simulink subsystem "MPC"  (R2024a)
settings: Solver=VariableStepAuto  StartTime=0.0  StopTime=10.0  RelTol=1e-3
libraries: mpclib x1
settings Model: Creator=cianc  LastModifiedBy=cianc

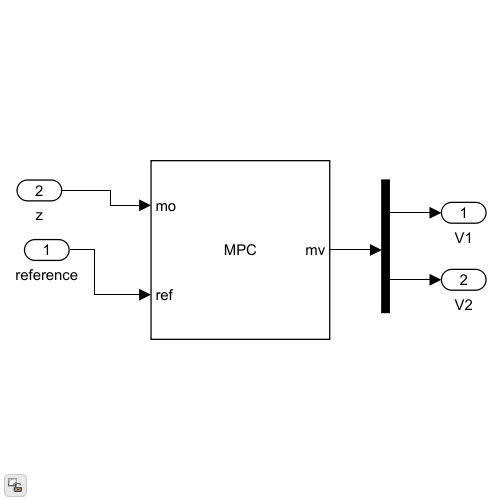
[thumbnail: Simulink's stored preview of the top-level diagram]
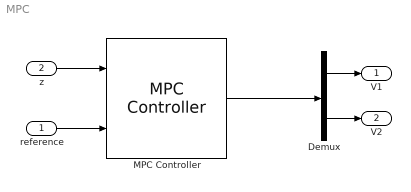
== system MPC ==
  reference : Inport
  z : Inport  Port=2
  Demux : Demux  Outputs=2
  MPC Controller : mpclib/MPC Controller  SCDEnableBlockLinearizationSpecification=on  is_multiple=0  enable_value=0  return_u0=off  updateMPCinCallerWorkspace=on  md_inport=off  mv_inport=off  uref_inport=off  return_cost=off  return_mvseq=off  return_qpstatus=off  return_xseq=off  return_state=off  return_ovseq=off  state_inport=off  umin_inport=off  umax_inport=off  ymin_inport=off  ymax_inport=off  cc_inport=off  ywt_inport=off  uwt_inport=off  duwt_inport=off  rhoeps_inport=off  pm_inport=off  MaximumP=10  HorizonChoice=FixedHorizon  n_ts=0.1  n_p=10  n_mv=2  n_md=1  n_ud=0  n_mo=1  n_uo=0  BlockDataType=double  SampleTimeInherited=off  switch_inport=off
  V1 : Outport
  V2 : Outport  Port=2
  wires:
  reference/1 -> MPC Controller/2
  z/1 -> MPC Controller/1
  Demux/1 -> V1/1
  Demux/2 -> V2/1
  MPC Controller/1 -> Demux/1
